simulink model "inverse_dynamics"  (R2021a)
settings: Solver=VariableStepAuto  StartTime=0.0  StopTime=10.0  RelTol=1e-3
values from neighbouring files (symbols this model uses):
  Kd = 10    [inverse_dynamics_script.m]
  Kp = 50    [inverse_dynamics_script.m]
libraries: roblocks x3
settings Model: Creator=root  LastModifiedBy=root

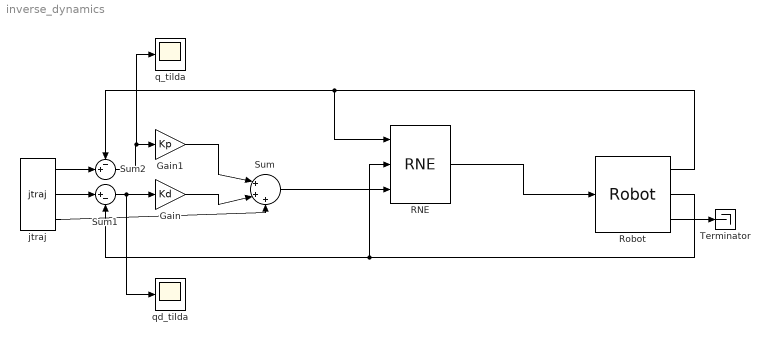
== system inverse_dynamics ==
  Gain : Gain  Gain=Kd
  Gain1 : Gain  Gain=Kp
  RNE : roblocks/Arm/RNE  robot=ur5  grav=[0 0 9.81]
  Robot : roblocks/Arm/Robot  robot=ur5  q0=[0 0 0 0 0 0]
  Sum : Sum  Inputs=|+++
  Sum1 : Sum  Inputs=|+-
  Sum2 : Sum  Inputs=-+|
  Terminator : Terminator
  jtraj : roblocks/Toolbox/jtraj  q0=[0 0 0 0 0 0]  qf=[pi/4 pi/2 -pi/2 0 0 0]  tmax=10  ts=0.02
  q_tilda : Scope
  qd_tilda : Scope
  wires:
  RNE/1 -> Robot/1
  jtraj/3 -> Sum/3
  jtraj/2 -> Sum1/1
  Robot/2 -> RNE/2, Sum1/2
  Sum1/1 -> qd_tilda/1, Gain/1
  Gain/1 -> Sum/2
  jtraj/1 -> Sum2/2
  Robot/1 -> RNE/1, Sum2/1
  Sum2/1 -> q_tilda/1, Gain1/1
  Gain1/1 -> Sum/1
  Sum/1 -> RNE/3
  Robot/3 -> Terminator/1
